simulink model "emulatedLift"  (R2020a)
settings: Solver=VariableStepAuto  StartTime=0.0  StopTime=10.0  RelTol=1e-3
undefined symbols (not defined in the file): sigbuilder_block
settings Model: Creator=DELL  LastModifiedBy=DELL

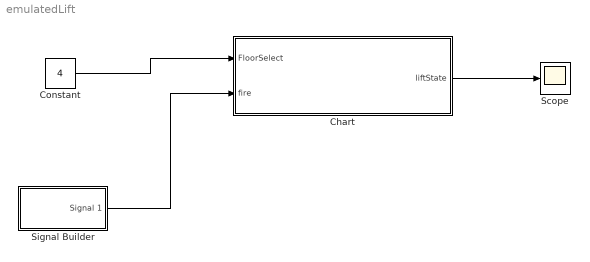
== system emulatedLift ==
  Chart : Stateflow chart  TreatAsAtomicUnit=on
  Constant : Constant  Value=4
  Scope : Scope
  Signal Builder : Subsystem  Tag=STV Subsys  LoadFcn=sigbuilder_block('load');  StartFcn=sigbuilder_block('start');  StopFcn=sigbuilder_block('stop');  ClipboardFcn=sigbuilder_block('clipboard');  mask(Sigbuilder block){tuvar=[0:10]}
      mask help: Simulink:masks:SigbuilderBlock_MD
      mask init:
      | if ~strcmp(get_param(bdroot(gcbh),'SimulationStatus'),'stopped') tuvar = sigbuilder_block('maskInit'); end
      settings: CopyFcn=sigbuilder_block('copy');  DeleteFcn=sigbuilder_block('delete');  ModelCloseFcn=sigbuilder_block('modelClose');  PreSaveFcn=sigbuilder_block('preSave');  PauseFcn=sigbuilder_block('pause');  ContinueFcn=sigbuilder_block('continue');  NameChangeFcn=sigbuilder_block('namechange');  OpenFcn=sigbuilder_block('open',[437.6 199.2 550.4 400 ]);  CloseFcn=sigbuilder_block('close');
      mask Display: plot(0, 0, 100, 100,[2, 2, 32, 32, 2], [68, 8, 8, 68, 68],[32, 2], [38, 38], [32, 19, 2],[53, 60, 44], [32, 17, 17, 2],[16, 16, 31, 31]);txt = getActiveGroup(gcbh);text(2, 100, txt,'verticalAlignment', 'top');
  wires:
  Constant/1 -> Chart/1(FloorSelect)
  Signal Builder/1(Signal 1) -> Chart/2(fire)
  Chart/1(liftState) -> Scope/1

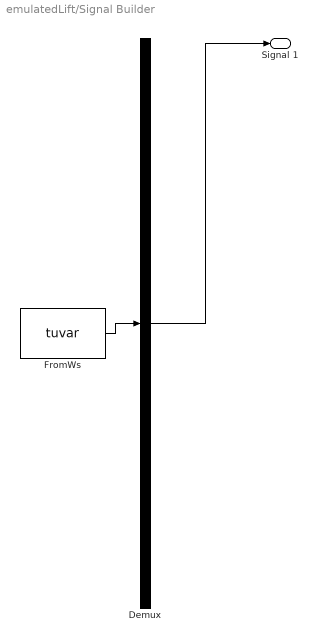
== system emulatedLift/Signal Builder ==
  Demux : Demux  Tag=STV Demux  Outputs=1
      settings: DisplayOption=none
  FromWs : FromWorkspace  Tag=STV FromWs  VariableName=tuvar
      SigBuilderData=|
      | common.afterFinalStr = 'Extrapolate'
      | common.sampleTime = 0
      | dataSet.timeRange = [0 10]
      | dataSet.name = 'Group 1'
      | sbobj.Groups.Name = 'Group 1'
      | sbobj.Groups.Signals.Name = 'Signal 1'
      | sbobj.Groups.Signals.XData = [0 4 4 6 6 10]
      | sbobj.Groups.Signals.YData = [0 0 1 1 0 0]
  Signal 1 : Outport  Tag=STV Outport
  wires:
  Demux/1 -> Signal 1/1
  FromWs/1 -> Demux/1

== stateflow chart emulatedLift/Chart ==
  state LiftOn
    en:
    liftState = 1;
    (history)
    state Floor0
      en:
      up = 0;down = 0
      cFloor = 0;
      movFloor(cFloor);
    state Floor1
      en:
      up = 0;down = 0
      cFloor = 1;
      movFloor(cFloor);
    state Floor2
      en:
      up = 0;down = 0
      cFloor = 2;
      movFloor(cFloor);
    state Floor3
      en:
      up = 0;down = 0
      cFloor = 3;
      movFloor(cFloor);
    state Floor4
      en:
      up = 0;down = 0
      cFloor = 4;
      movFloor(cFloor);
    state Floor5
      en:
      up = 0;down = 0
      cFloor = 5;
      movFloor(cFloor);
    (default) -> Floor0
    Floor0 -> Floor1 : [up == 1]
    Floor1 -> Floor0 [order 1] : [down == 1]
    Floor2 -> Floor1 [order 1] : [down ==1]
    Floor1 -> Floor2 [order 2] : [up == 1]
    Floor3 -> Floor2 [order 1] : [down ==1]
    Floor2 -> Floor3 [order 2] : [up ==1]
    Floor3 -> Floor4 [order 2] : [up ==1]
    Floor4 -> Floor3 [order 1] : [down == 1]
    Floor4 -> Floor5 [order 2] : [up ==1]
    Floor5 -> Floor4 : [down ==1]
  state y = movFloor(floor) [function]
    (default) -> (junction 64) : % move floor
    (junction 64) -> (junction 65) [order 1] : [FloorSelect > floor]
    (junction 64) -> (junction 66) [order 2]
    (junction 65) -> (junction 70) : {up = 1;}
    (junction 66) -> (junction 67) [order 1] : [FloorSelect < floor]
    (junction 66) -> (junction 68) [order 2]
    (junction 67) -> (junction 69) : {down =1;}
    (junction 69) -> (junction 68)
    (junction 70) -> (junction 69)
    (junction 68) -> (junction 71)
  state LiftOff
    en:
    liftState = 0;
  (default) -> LiftOn
  LiftOn -> LiftOff : [fire ==1]
  LiftOff -> LiftOn : [fire ==0]
  data: floor function_input; y function_output; up local; down local; cFloor local; FloorSelect input; liftState output; fire input
